simulink model "diff_eq"  (R2022b)
settings: Solver=VariableStepAuto  StartTime=0.0  StopTime=10.0  RelTol=1e-3
undefined symbols (not defined in the file or in its folder): a1, a2, a3, b1, b2, b3, c1, c2, c3, k1, k2, k3
settings Model: Creator=Brigosha_Guest  LastModifiedBy=Brigosha_Guest

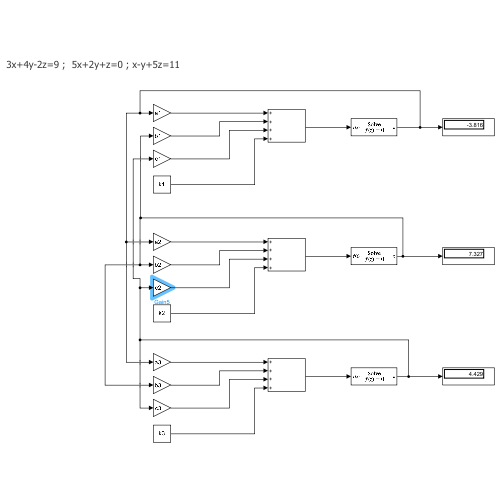
[thumbnail: Simulink's stored preview of the top-level diagram]
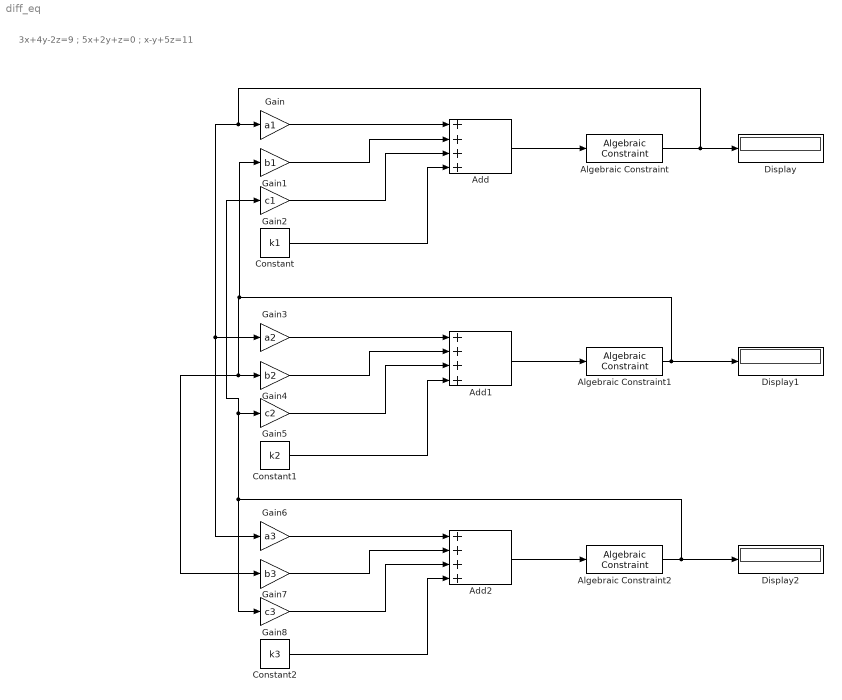
== system diff_eq ==
  note: 3x+4y-2z=9 ; 5x+2y+z=0 ; x-y+5z=11
  Add : Sum  Inputs=++++
  Add1 : Sum  Inputs=++++
  Add2 : Sum  Inputs=++++
  Algebraic Constraint : AlgebraicConstraint
  Algebraic Constraint1 : AlgebraicConstraint
  Algebraic Constraint2 : AlgebraicConstraint
  Constant : Constant  Value=k1
  Constant1 : Constant  Value=k2
  Constant2 : Constant  Value=k3
  Display : Display
  Display1 : Display
  Display2 : Display
  Gain : Gain  Gain=a1
  Gain1 : Gain  Gain=b1
  Gain2 : Gain  Gain=c1
  Gain3 : Gain  Gain=a2
  Gain4 : Gain  Gain=b2
  Gain5 : Gain  Gain=c2
  Gain6 : Gain  Gain=a3
  Gain7 : Gain  Gain=b3
  Gain8 : Gain  Gain=c3
  wires:
  Gain/1 -> Add/1
  Algebraic Constraint/1 -> Gain/1, Gain6/1, Gain3/1, Display/1
  Add/1 -> Algebraic Constraint/1
  Constant/1 -> Add/4
  Gain1/1 -> Add/2
  Gain2/1 -> Add/3
  Gain5/1 -> Add1/3
  Gain4/1 -> Add1/2
  Constant1/1 -> Add1/4
  Add1/1 -> Algebraic Constraint1/1
  Algebraic Constraint1/1 -> Gain1/1, Gain7/1, Gain4/1, Display1/1
  Gain3/1 -> Add1/1
  Gain6/1 -> Add2/1
  Algebraic Constraint2/1 -> Gain8/1, Gain2/1, Gain5/1, Display2/1
  Add2/1 -> Algebraic Constraint2/1
  Constant2/1 -> Add2/4
  Gain7/1 -> Add2/2
  Gain8/1 -> Add2/3
